simulink model "sv1_0"  (R2022b)
settings: Solver=VariableStepAuto  StartTime=0.0  StopTime=10.0  RelTol=1e-3
values from neighbouring files (symbols this model uses):
  m = rotation_matrix([0 0 1], theta)    [ectopic.m]    (also in ectopic_dirty_1.m; workspace.m)
undefined symbols (not defined in the file or in its folder): X, Y, Z
libraries: sm_lib x67, nesl_utility x1
(part 2 of 2)

== matlab function sv1_0/杆件的偏角速度、偏速度矩阵/偏角速度矩阵与偏速度矩阵2 ==
  data: L input; n input; S input; J input; O2 output; V2 output
function [O2,V2]=fcn(L,n,S,J)
OO1=zeros(1,6);
E=eye(3,3);
s=skew(S(:,2));%求反对称矩阵
OO3=J(2,:);
OO4=[OO1;OO1;OO3];
O2=skew((n(:,2)/L))*([E,s]-OO4);%杆件偏角速度
V2=OO4-L/2*skew((n(:,2)))*O2;%杆件偏速度

== matlab function sv1_0/杆件的偏角速度、偏速度矩阵/偏角速度矩阵与偏速度矩阵3 ==
  data: L input; n input; S input; J input; O3 output; V3 output
function [O3,V3]=fcn(L,n,S,J)
OO1=zeros(1,6);
E=eye(3,3);
s=skew(S(:,3));%求反对称矩阵
OO3=J(3,:);
OO4=[OO1;OO1;OO3];
O3=skew((n(:,3)/L))*([E,s]-OO4);%杆件偏角速度
V3=OO4-L/2*skew((n(:,3)))*O3;%杆件偏速度
